simulink model "fir_t1"  (R2017a)
settings: Solver=VariableStepAuto  StartTime=0.0  StopTime=120  RelTol=1e-3
settings Model: Creator=Chaohua Zhao  LastModifiedBy=Chaohua Zhao

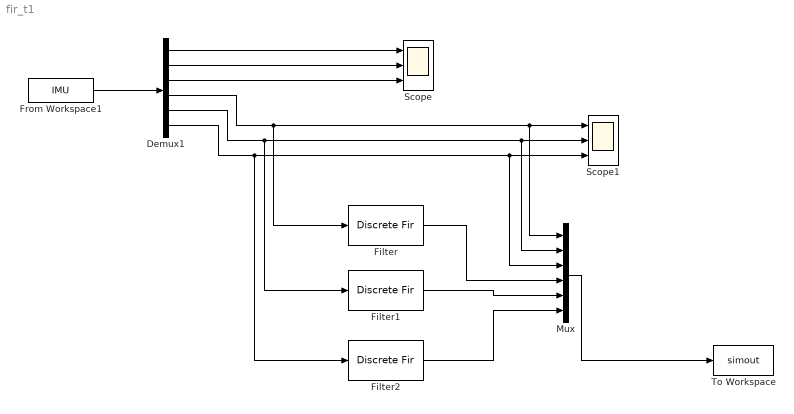
== system fir_t1 ==
  Demux1 : Demux  Outputs=6
  Filter : DiscreteFir  Tag=BlockMethodSubSystem  Coefficients=[0 0.0054786758595111026 0.042763636162144819 0.12151889269739169 0.20757905037865335 0.245319489804598 0.20757905037865335 0.12151889269739169 0.042763636162144819 0.0054786758595111026 0]  InputProcessing=Columns as channels (frame based)
  Filter1 : DiscreteFir  Tag=BlockMethodSubSystem  Coefficients=[0 0.0054786758595111026 0.042763636162144819 0.12151889269739169 0.20757905037865335 0.245319489804598 0.20757905037865335 0.12151889269739169 0.042763636162144819 0.0054786758595111026 0]  InputProcessing=Columns as channels (frame based)
  Filter2 : DiscreteFir  Tag=BlockMethodSubSystem  Coefficients=[0 0.0054786758595111026 0.042763636162144819 0.12151889269739169 0.20757905037865335 0.245319489804598 0.20757905037865335 0.12151889269739169 0.042763636162144819 0.0054786758595111026 0]  InputProcessing=Columns as channels (frame based)
  From Workspace1 : FromWorkspace  VariableName=IMU  SampleTime=0.003  OutputAfterFinalValue=Setting to zero
  Mux : Mux  Inputs=6
  Scope : Scope  NumInputPorts=3
  Scope1 : Scope  NumInputPorts=3
  To Workspace : ToWorkspace  VariableName=simout  SampleTime=-1
  wires:
  From Workspace1/1 -> Demux1/1
  Demux1/1 -> Scope/1
  Demux1/2 -> Scope/2
  Demux1/3 -> Scope/3
  Demux1/4 -> Filter/1, Mux/1, Scope1/1
  Demux1/5 -> Filter1/1, Mux/2, Scope1/2
  Demux1/6 -> Filter2/1, Mux/3, Scope1/3
  Mux/1 -> To Workspace/1
  Filter/1 -> Mux/4
  Filter1/1 -> Mux/5
  Filter2/1 -> Mux/6
